simulink model "Test_Bit_Multiplexer_8_to_1"  (Simulink 8.1)
settings: Solver=ode45  StartTime=0.0  StopTime=len  RelTol=1e-3
libraries: commutil2 x2, Bit_Multiplexers_Lib x1
settings Model: Creator=N  LastModifiedBy=uzivatel
settings DataIOCC: LimitDataPoints=off  SignalLoggingSaveFormat=Dataset
settings OptimizationCC: ExpressionDepthLimit=128
settings DebuggingCC: UnderspecifiedInitializationDetection=Simplified  MergeDetectMultiDrivingBlocksExec=error  SolverPrmCheckMsg=none  FcnCallInpInsideContextMsg=EnableAllAsError  FrameProcessingCompatibilityMsg=error  StateNameClashWarn=none
settings HardwareCC: ProdBitPerPointer=64  ProdLargestAtomicFloat=Float  ProdIntDivRoundTo=Zero  ProdEndianess=LittleEndian  ProdHWDeviceType=Intel->x86-64 (Windows64)
settings ModelReferenceCC: PropagateSignalLabelsOutOfModel=on
settings GRTTargetCC: CodeReplacementLibrary=None  CombineOutputUpdateFcns=on  CPPClassGenCompliant=on  GRTInterface=off

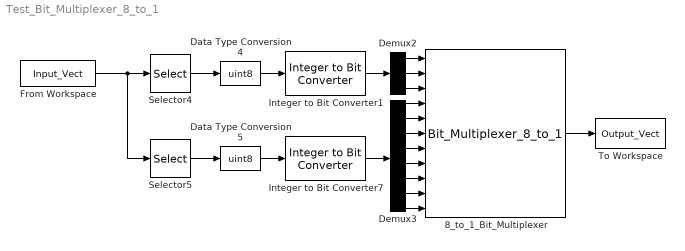
== system Test_Bit_Multiplexer_8_to_1 ==
  8_to_1_Bit_Multiplexer : Bit_Multiplexers_Lib/Bit_Multiplexers_Lib/Bit_Multiplexer_8_to_1
  Data Type Conversion4 : DataTypeConversion  OutDataTypeStr=uint8
  Data Type Conversion5 : DataTypeConversion  OutDataTypeStr=uint8
  Demux2 : Demux  Outputs=3
  Demux3 : Demux  Outputs=8
  From Workspace : FromWorkspace  VariableName=Input_Vect  SampleTime=1  Interpolate=off  OutputAfterFinalValue=Holding final value
  Integer to Bit Converter1 : commutil2/Integer to Bit Converter  nbits=3  signedInputValues=Unsigned  bitOrder=MSB first  outDtype=boolean
  Integer to Bit Converter7 : commutil2/Integer to Bit Converter  nbits=8  signedInputValues=Unsigned  bitOrder=MSB first  outDtype=uint8
  Selector4 : Selector  IndexMode=Zero-based  InputPortWidth=2  SampleTime=1  IndexOptions=Index vector (dialog)  Indices=0  OutputSizes=1
  Selector5 : Selector  IndexMode=Zero-based  InputPortWidth=2  IndexOptions=Index vector (dialog)  Indices=1  OutputSizes=1
  To Workspace : ToWorkspace  VariableName=Output_Vect  SampleTime=1
  wires:
  Demux2/1 -> 8_to_1_Bit_Multiplexer/1
  Demux2/2 -> 8_to_1_Bit_Multiplexer/2
  Demux2/3 -> 8_to_1_Bit_Multiplexer/3
  Integer to Bit Converter1/1 -> Demux2/1
  Demux3/1 -> 8_to_1_Bit_Multiplexer/4
  Demux3/2 -> 8_to_1_Bit_Multiplexer/5
  Demux3/3 -> 8_to_1_Bit_Multiplexer/6
  Demux3/4 -> 8_to_1_Bit_Multiplexer/7
  Demux3/5 -> 8_to_1_Bit_Multiplexer/8
  Demux3/6 -> 8_to_1_Bit_Multiplexer/9
  Demux3/7 -> 8_to_1_Bit_Multiplexer/10
  Demux3/8 -> 8_to_1_Bit_Multiplexer/11
  From Workspace/1 -> Selector5/1, Selector4/1
  Selector4/1 -> Data Type Conversion4/1
  Selector5/1 -> Data Type Conversion5/1
  Data Type Conversion4/1 -> Integer to Bit Converter1/1
  Data Type Conversion5/1 -> Integer to Bit Converter7/1
  8_to_1_Bit_Multiplexer/1 -> To Workspace/1
  Integer to Bit Converter7/1 -> Demux3/1
